simulink model "mode_controller"  (R2017a)
settings: Solver=VariableStepAuto  StartTime=0.0  StopTime=10  RelTol=1e-3
settings Model: Creator=mini  LastModifiedBy=mini
settings OptimizationCC: DefaultParameterBehavior=Inlined

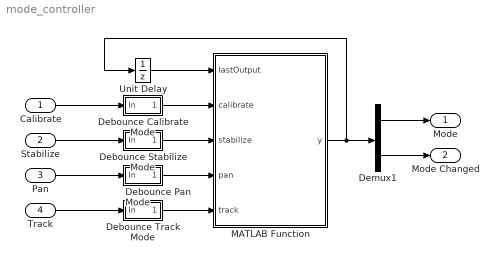
== system mode_controller ==
  Calibrate : Inport
  Stabilize : Inport  Port=2
  Pan : Inport  Port=3
  Track : Inport  Port=4
  Debounce Calibrate Mode : Subsystem  TreatAsAtomicUnit=on  mask(Debounce){debounce_count=20}
      mask prompts: debounce_count "Debounce count"
      mask help: Number of consecutive samples before changing states.
  Debounce Pan Mode : Subsystem  TreatAsAtomicUnit=on  mask(Debounce){debounce_count=20}
      mask prompts: debounce_count "Debounce count"
      mask help: Number of consecutive samples before changing states.
  Debounce Stabilize Mode : Subsystem  TreatAsAtomicUnit=on  mask(Debounce){debounce_count=20}
      mask prompts: debounce_count "Debounce count"
      mask help: Number of consecutive samples before changing states.
  Debounce Track Mode : Subsystem  TreatAsAtomicUnit=on  mask(Debounce){debounce_count=20}
      mask prompts: debounce_count "Debounce count"
      mask help: Number of consecutive samples before changing states.
  Demux1 : Demux  Outputs=2
  MATLAB Function : MATLAB Function  TreatAsAtomicUnit=on
  Unit Delay : UnitDelay  SampleTime=-1
  Mode : Outport
  Mode Changed : Outport  Port=2
  wires:
  Debounce Stabilize Mode/1(Out) -> MATLAB Function/3(stabilize)
  Stabilize/1 -> Debounce Stabilize Mode/1(In)
  Pan/1 -> Debounce Pan Mode/1(In)
  Debounce Pan Mode/1(Out) -> MATLAB Function/4(pan)
  Demux1/1 -> Mode/1
  Calibrate/1 -> Debounce Calibrate Mode/1(In)
  Debounce Calibrate Mode/1(Out) -> MATLAB Function/2(calibrate)
  MATLAB Function/1(y) -> Unit Delay/1, Demux1/1
  Track/1 -> Debounce Track Mode/1(In)
  Unit Delay/1 -> MATLAB Function/1(lastOutput)
  Debounce Track Mode/1(Out) -> MATLAB Function/5(track)
  Demux1/2 -> Mode Changed/1

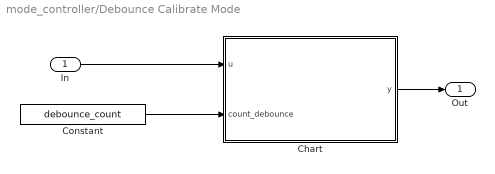
== system mode_controller/Debounce Calibrate Mode ==
  In : Inport
  Chart : Stateflow chart  TreatAsAtomicUnit=on
  Constant : Constant  Value=debounce_count  OutDataTypeStr=uint8  SampleTime=-1
  Out : Outport
  wires:
  In/1 -> Chart/1(u)
  Chart/1(y) -> Out/1
  Constant/1 -> Chart/2(count_debounce)

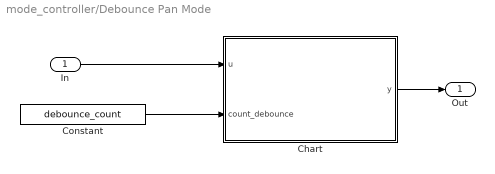
== system mode_controller/Debounce Pan Mode ==
  In : Inport
  Chart : Stateflow chart  TreatAsAtomicUnit=on
  Constant : Constant  Value=debounce_count  OutDataTypeStr=uint8  SampleTime=-1
  Out : Outport
  wires:
  In/1 -> Chart/1(u)
  Chart/1(y) -> Out/1
  Constant/1 -> Chart/2(count_debounce)

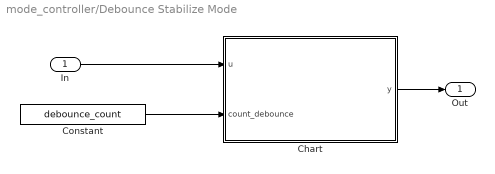
== system mode_controller/Debounce Stabilize Mode ==
  In : Inport
  Chart : Stateflow chart  TreatAsAtomicUnit=on
  Constant : Constant  Value=debounce_count  OutDataTypeStr=uint8  SampleTime=-1
  Out : Outport
  wires:
  In/1 -> Chart/1(u)
  Chart/1(y) -> Out/1
  Constant/1 -> Chart/2(count_debounce)

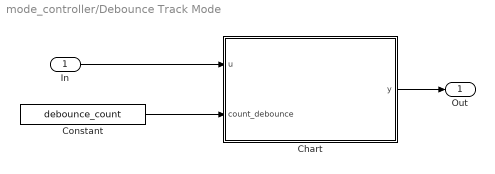
== system mode_controller/Debounce Track Mode ==
  In : Inport
  Chart : Stateflow chart  TreatAsAtomicUnit=on
  Constant : Constant  Value=debounce_count  OutDataTypeStr=uint8  SampleTime=-1
  Out : Outport
  wires:
  In/1 -> Chart/1(u)
  Chart/1(y) -> Out/1
  Constant/1 -> Chart/2(count_debounce)

== stateflow chart mode_controller/Debounce Calibrate Mode/Chart ==
  settings: executeAtInitialization=1
  (default) -> (junction 2)
  (junction 2) -> (junction 3) [order 1] : [u == u_n1]
  (junction 2) -> (junction 13) [order 2] : {count = 0;}
  (junction 3) -> (junction 5)
  (junction 5) -> (junction 7) [order 1] : [count >= count_debounce]
  (junction 7) -> (junction 9) : {y = u;}
  (junction 5) -> (junction 11) [order 2] : {count = count + 1;}
  (junction 11) -> (junction 13)
  (junction 9) -> (junction 11)
  (junction 13) -> (junction 17) : {u_n1 = u;}
  data: u input; u_n1 local type(u); y output type(u); count local uint8; count_debounce input

== stateflow chart mode_controller/Debounce Pan Mode/Chart ==
  settings: executeAtInitialization=1
  (default) -> (junction 2)
  (junction 2) -> (junction 3) [order 1] : [u == u_n1]
  (junction 2) -> (junction 13) [order 2] : {count = 0;}
  (junction 3) -> (junction 5)
  (junction 5) -> (junction 7) [order 1] : [count >= count_debounce]
  (junction 7) -> (junction 9) : {y = u;}
  (junction 5) -> (junction 11) [order 2] : {count = count + 1;}
  (junction 11) -> (junction 13)
  (junction 9) -> (junction 11)
  (junction 13) -> (junction 17) : {u_n1 = u;}
  data: u input; u_n1 local type(u); y output type(u); count local uint8; count_debounce input

== stateflow chart mode_controller/Debounce Stabilize Mode/Chart ==
  settings: executeAtInitialization=1
  (default) -> (junction 2)
  (junction 2) -> (junction 3) [order 1] : [u == u_n1]
  (junction 2) -> (junction 13) [order 2] : {count = 0;}
  (junction 3) -> (junction 5)
  (junction 5) -> (junction 7) [order 1] : [count >= count_debounce]
  (junction 7) -> (junction 9) : {y = u;}
  (junction 5) -> (junction 11) [order 2] : {count = count + 1;}
  (junction 11) -> (junction 13)
  (junction 9) -> (junction 11)
  (junction 13) -> (junction 17) : {u_n1 = u;}
  data: u input; u_n1 local type(u); y output type(u); count local uint8; count_debounce input

== stateflow chart mode_controller/Debounce Track Mode/Chart ==
  settings: executeAtInitialization=1
  (default) -> (junction 2)
  (junction 2) -> (junction 3) [order 1] : [u == u_n1]
  (junction 2) -> (junction 13) [order 2] : {count = 0;}
  (junction 3) -> (junction 5)
  (junction 5) -> (junction 7) [order 1] : [count >= count_debounce]
  (junction 7) -> (junction 9) : {y = u;}
  (junction 5) -> (junction 11) [order 2] : {count = count + 1;}
  (junction 11) -> (junction 13)
  (junction 9) -> (junction 11)
  (junction 13) -> (junction 17) : {u_n1 = u;}
  data: u input; u_n1 local type(u); y output type(u); count local uint8; count_debounce input

== matlab function mode_controller/MATLAB Function ==
  data: lastOutput input; y output; calibrate input; stabilize input; pan input; track input
function y = fcn(lastOutput, calibrate, stabilize, pan, track)
    % default action on startup 
    % possible TODO add OFF mode
    
    % won't happen on startup
    if( isvector(lastOutput) && length(lastOutput) == 2 )
        lastMode = lastOutput(1);
        lastUpdated = lastOutput(2);
    else
        % set default mode on startup
        lastMode = 1;
        lastUpdated = 0;
    end
    % change mode based on inputs
    if ( calibrate || lastMode == 0 )
        mode = 1;
    elseif ( stabilize )
        mode = 2;
    elseif ( pan )
        mode = 3;
    elseif ( track )
        mode = 4;
    else
        mode = lastMode;
    end
    % trigger update if mode just changed
    if ( mode ~= lastMode && lastUpdated ~= 1 )
        updated = 1;
    else
        updated = 0;
    end
y = [mode, updated];
